simulink model "HyL"  (R2015b)
settings: Solver=ode23  StartTime=0.0  StopTime=1  FixedStep=1e-4  RelTol=1e-3  AbsTol=1e-4
undefined symbols (not defined in the file): a1, a2, Aa, Ab, b1, b2, base, beta, fv, hipassembly, In, KI, KP, Kva, Kvb, KvlkA, KvlkB, L, Lcyl, leak, lowerleg, lw_dz, pAo, pBo, ps, pt, sup1, up_dz, upperleg, V0A, V0B, wn
libraries: mblibv1 x22, simulink x6
settings Model: Creator=Toshiba  LastModifiedBy=Toshiba
settings SolverCC: ZeroCrossAlgorithm=Adaptive  SolverResetMethod=Robust
settings DataIOCC: OutputTimes=[0:1/30:100]
settings SimMechanicsCC: VisOnUpdateDiagram=on  VisDuringSimulation=on

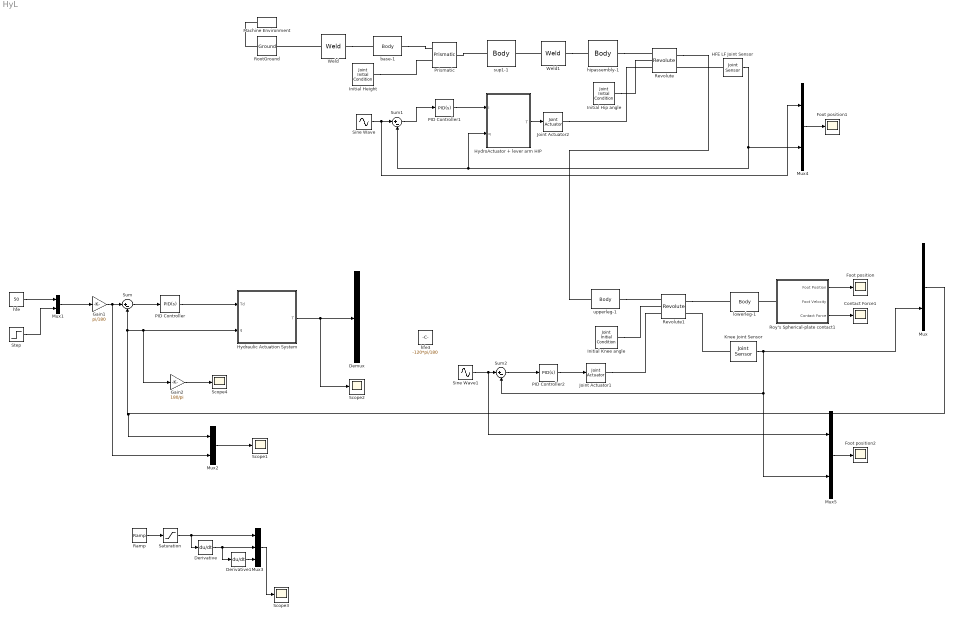
== system HyL ==
  Contact Force1 : Scope
  Demux : Demux  Outputs=2
  Derivative : Derivative
  Derivative1 : Derivative
  Foot position : Scope
  Foot position1 : Scope
  Foot position2 : Scope
  Gain1 : Gain  Gain=pi/180
  Gain2 : Gain  Gain=180/pi
  HFE LF Joint Sensor : mblibv1/Sensors &  Actuators/Joint Sensor  UpdateFromCAD=off  PhysicalDomain=Mechanical  PortType=blob  Muxed=off  Pose=off  Angle=on  AngleUnits=rad  ArcVelocity=off  ArcVelocityUnits=rad/s  ArcAcceleration=off  ArcAccelerationUnits=rad/s^2  CoordPosition=on  CoordPositionUnits=m  Velocity=off  VelocityUnits=m/s  Acceleration=off  AccelerationUnits=m/s^2  Quaternion=on  QuaternionDT=off  QuaternionDDT=off  QuaternionUnits=off  OutputVector=[ 1 ]  ActiveIO=on  Width=1  DialogClass=MechanicalSensorBlock  Primitive=R1  Force=off  ForceUnits=N  Torque=off  TorqueUnits=N*m  ReferenceFrame=Absolute (INERTIAL)  ReactionSensedSide=Base  ReactionReferenceFrame=Absolute (World)  ReactionForce=off  ReactionForceUnits=N  ReactionMoment=off  ReactionMomentUnits=N*m
  Hydraulic Actuation System : Subsystem
  HydroActuator + lever arm HIP : Subsystem
  Initial Height : mblibv1/Sensors &  Actuators/Joint Initial Condition  UpdateFromCAD=off  LeftPortType=blob  RightPortType=blob  PhysicalDomain=Mechanical  DialogClass=InitialConditionBlock  InitialConditions=P1$true$0$m$rad$0$m/s$rad/s#P2$false$0$m$rad$0$m/s$rad/s#P3$false$0$m$rad$0$m/s$rad/s#R1$false$0$m$rad$0$m/s$rad/s#R2$false$0$m$rad$0$m/s$rad/s#R3$false$0$m$rad$0$m/s$rad/s#S$false$0$m$rad$0$m/s$rad/s  P1PIC=0  P1VIC=0  P2PIC=0  P2VIC=0  P3PIC=0  P3VIC=0  R1PIC=0  R1VIC=0  R2PIC=0  R2VIC=0  R3PIC=0  R3VIC=0  SPIC=0  SVIC=0
  Initial Hip angle : mblibv1/Sensors &  Actuators/Joint Initial Condition  UpdateFromCAD=off  LeftPortType=blob  RightPortType=blob  PhysicalDomain=Mechanical  DialogClass=InitialConditionBlock  InitialConditions=P1$false$0.7$m$rad$0$m/s$rad/s#P2$false$0$m$rad$0$m/s$rad/s#P3$false$0$m$rad$0$m/s$rad/s#R1$true$45$m$deg$0$m/s$rad/s#R2$false$0$m$rad$0$m/s$rad/s#R3$false$0$m$rad$0$m/s$rad/s#S$false$0$m$rad$0$m/s$rad/s  P1PIC=0  P1VIC=0  P2PIC=0  P2VIC=0  P3PIC=0  P3VIC=0  R1PIC=45  R1VIC=0  R2PIC=0  R2VIC=0  R3PIC=0  R3VIC=0  SPIC=0  SVIC=0
  Initial Knee angle : mblibv1/Sensors &  Actuators/Joint Initial Condition  UpdateFromCAD=off  LeftPortType=blob  RightPortType=blob  PhysicalDomain=Mechanical  DialogClass=InitialConditionBlock  InitialConditions=P1$false$0.7$m$rad$0$m/s$rad/s#P2$false$0$m$rad$0$m/s$rad/s#P3$false$0$m$rad$0$m/s$rad/s#R1$true$-90$m$deg$0$m/s$rad/s#R2$false$0$m$rad$0$m/s$rad/s#R3$false$0$m$rad$0$m/s$rad/s#S$false$0$m$rad$0$m/s$rad/s  P1PIC=0  P1VIC=0  P2PIC=0  P2VIC=0  P3PIC=0  P3VIC=0  R1PIC=-90  R1VIC=0  R2PIC=0  R2VIC=0  R3PIC=0  R3VIC=0  SPIC=0  SVIC=0
  Joint Actuator1 : mblibv1/Sensors &  Actuators/Joint Actuator  UpdateFromCAD=off  PhysicalDomain=Mechanical  PortType=blob  ActuationStyle=Force  AngleUnits=deg  ArcVelocityUnits=deg/s  ArcAccelerationUnits=deg/s^2  CoordPositionUnits=m  VelocityUnits=m/s  AccelerationUnits=m/s^2  ForceUnits=N  TorqueUnits=N*m  ActiveIO=on  Width=1  DialogClass=MechanicalActuatorBlock  Primitive=R1  ReferenceFrame=Absolute (World)
  Joint Actuator2 : mblibv1/Sensors &  Actuators/Joint Actuator  UpdateFromCAD=off  PhysicalDomain=Mechanical  PortType=blob  ActuationStyle=Force  AngleUnits=deg  ArcVelocityUnits=deg/s  ArcAccelerationUnits=deg/s^2  CoordPositionUnits=m  VelocityUnits=m/s  AccelerationUnits=m/s^2  ForceUnits=N  TorqueUnits=N*m  ActiveIO=on  Width=1  DialogClass=MechanicalActuatorBlock  Primitive=R1  ReferenceFrame=Absolute (World)
  Knee Joint Sensor : mblibv1/Sensors &  Actuators/Joint Sensor  UpdateFromCAD=off  PhysicalDomain=Mechanical  PortType=blob  Muxed=off  Pose=off  Angle=on  AngleUnits=rad  ArcVelocity=off  ArcVelocityUnits=rad/s  ArcAcceleration=off  ArcAccelerationUnits=rad/s^2  CoordPosition=on  CoordPositionUnits=m  Velocity=off  VelocityUnits=m/s  Acceleration=off  AccelerationUnits=m/s^2  Quaternion=on  QuaternionDT=off  QuaternionDDT=off  QuaternionUnits=off  OutputVector=[ 1 ]  ActiveIO=on  Width=1  DialogClass=MechanicalSensorBlock  Primitive=R1  Force=off  ForceUnits=N  Torque=off  TorqueUnits=N*m  ReferenceFrame=Absolute (INERTIAL)  ReactionSensedSide=Base  ReactionReferenceFrame=Absolute (World)  ReactionForce=off  ReactionForceUnits=N  ReactionMoment=off  ReactionMomentUnits=N*m
  Machine Environment : mblibv1/Bodies/Machine Environment  PortType=env  PhysicalDomain=Mechanical  DialogTemplateClass=MECH.MachineEnvironment  SyncWhenCopied=off  Gravity=[0 -9.81 0]  GravityUnits=m/s^2  GravityAsSignal=off  Dimensionality=Auto-detect  AnalysisType=Forward dynamics  LinearAssemblyTolerance=1e-3  LinearAssemblyToleranceUnits=m  AngularAssemblyTolerance=1e-3  AngularAssemblyToleranceUnits=rad  ConstraintSolverType=Stabilizing  ConstraintRelTolerance=1e-4  ConstraintAbsTolerance=1e-4  UseRobustSingularityHandling=off  RedundancyAnalysisToleranceType=Automatically select tolerance  RedundancyAnalysisTolerance=1e-14  StatePerturbationType=Fixed  PerturbationSize=1e-5  VisualizeMachine=on  BodyVisualizationType=Use model default body geometries  BodyColorSelMode=Use model default  DefaultBodyColor=[1 0 0]
  Mux{,1..2,4..5} (5 alike) : Mux  Inputs=2
  Mux3 : Mux  Inputs=3
  PID Controller : simulink/Continuous/PID Controller  Controller=PID  TimeDomain=Continuous-time  SampleTime=-1  IntegratorMethod=Forward Euler  FilterMethod=Forward Euler  Form=Parallel  UseFilter=on  ControllerParametersSource=internal  P=200  I=0  D=6  N=100  InitialConditionSource=internal  InitialConditionForIntegrator=0  InitialConditionForFilter=0  ExternalReset=none  LimitOutput=off  UpperSaturationLimit=inf  LowerSaturationLimit=-inf  LinearizeAsGain=on  AntiWindupMode=none  Kb=1  TrackingMode=off  Kt=1  PParamMin=[]  PParamMax=[]  IParamMin=[]  IParamMax=[]  DParamMin=[]  DParamMax=[]  NParamMin=[]  NParamMax=[]  KbParamMin=[]  KbParamMax=[]  KtParamMin=[]  KtParamMax=[]  POutMin=[]  POutMax=[]  IOutMin=[]  IOutMax=[]  DOutMin=[]  DOutMax=[]  NOutMin=[]  NOutMax=[]  KbOutMin=[]  KbOutMax=[]  KtOutMin=[]  KtOutMax=[]  IntegratorOutMin=[]  IntegratorOutMax=[]  FilterOutMin=[]  FilterOutMax=[]  SumOutMin=[]  SumOutMax=[]  SumI1OutMin=[]  SumI1OutMax=[]  SumI2OutMin=[]  SumI2OutMax=[]  SumI3OutMin=[]  SumI3OutMax=[]  SumDOutMin=[]  SumDOutMax=[]  SaturationOutMin=[]  SaturationOutMax=[]  IntegratorContinuousStateAttributes=''  IntegratorStateMustResolveToSignalObject=off  IntegratorRTWStateStorageClass=Auto  FilterContinuousStateAttributes=''  FilterStateMustResolveToSignalObject=off  FilterRTWStateStorageClass=Auto  DifferentiatorICPrevScaledInput=0  DifferentiatorOutMin=[]  DifferentiatorOutMax=[]
  PID Controller1 : simulink/Continuous/PID Controller  Controller=PID  TimeDomain=Continuous-time  SampleTime=-1  IntegratorMethod=Forward Euler  FilterMethod=Forward Euler  Form=Parallel  UseFilter=on  ControllerParametersSource=internal  P=300  I=0  D=6  N=100  InitialConditionSource=internal  InitialConditionForIntegrator=0  InitialConditionForFilter=0  ExternalReset=none  LimitOutput=off  UpperSaturationLimit=inf  LowerSaturationLimit=-inf  LinearizeAsGain=on  AntiWindupMode=none  Kb=1  TrackingMode=off  Kt=1  PParamMin=[]  PParamMax=[]  IParamMin=[]  IParamMax=[]  DParamMin=[]  DParamMax=[]  NParamMin=[]  NParamMax=[]  KbParamMin=[]  KbParamMax=[]  KtParamMin=[]  KtParamMax=[]  POutMin=[]  POutMax=[]  IOutMin=[]  IOutMax=[]  DOutMin=[]  DOutMax=[]  NOutMin=[]  NOutMax=[]  KbOutMin=[]  KbOutMax=[]  KtOutMin=[]  KtOutMax=[]  IntegratorOutMin=[]  IntegratorOutMax=[]  FilterOutMin=[]  FilterOutMax=[]  SumOutMin=[]  SumOutMax=[]  SumI1OutMin=[]  SumI1OutMax=[]  SumI2OutMin=[]  SumI2OutMax=[]  SumI3OutMin=[]  SumI3OutMax=[]  SumDOutMin=[]  SumDOutMax=[]  SaturationOutMin=[]  SaturationOutMax=[]  IntegratorContinuousStateAttributes=''  IntegratorStateMustResolveToSignalObject=off  IntegratorRTWStateStorageClass=Auto  FilterContinuousStateAttributes=''  FilterStateMustResolveToSignalObject=off  FilterRTWStateStorageClass=Auto  DifferentiatorICPrevScaledInput=0  DifferentiatorOutMin=[]  DifferentiatorOutMax=[]
  PID Controller2 : simulink/Continuous/PID Controller  Controller=PID  TimeDomain=Continuous-time  SampleTime=-1  IntegratorMethod=Forward Euler  FilterMethod=Forward Euler  Form=Parallel  UseFilter=on  ControllerParametersSource=internal  P=300  I=0  D=6  N=100  InitialConditionSource=internal  InitialConditionForIntegrator=0  InitialConditionForFilter=0  ExternalReset=none  LimitOutput=off  UpperSaturationLimit=inf  LowerSaturationLimit=-inf  LinearizeAsGain=on  AntiWindupMode=none  Kb=1  TrackingMode=off  Kt=1  PParamMin=[]  PParamMax=[]  IParamMin=[]  IParamMax=[]  DParamMin=[]  DParamMax=[]  NParamMin=[]  NParamMax=[]  KbParamMin=[]  KbParamMax=[]  KtParamMin=[]  KtParamMax=[]  POutMin=[]  POutMax=[]  IOutMin=[]  IOutMax=[]  DOutMin=[]  DOutMax=[]  NOutMin=[]  NOutMax=[]  KbOutMin=[]  KbOutMax=[]  KtOutMin=[]  KtOutMax=[]  IntegratorOutMin=[]  IntegratorOutMax=[]  FilterOutMin=[]  FilterOutMax=[]  SumOutMin=[]  SumOutMax=[]  SumI1OutMin=[]  SumI1OutMax=[]  SumI2OutMin=[]  SumI2OutMax=[]  SumI3OutMin=[]  SumI3OutMax=[]  SumDOutMin=[]  SumDOutMax=[]  SaturationOutMin=[]  SaturationOutMax=[]  IntegratorContinuousStateAttributes=''  IntegratorStateMustResolveToSignalObject=off  IntegratorRTWStateStorageClass=Auto  FilterContinuousStateAttributes=''  FilterStateMustResolveToSignalObject=off  FilterRTWStateStorageClass=Auto  DifferentiatorICPrevScaledInput=0  DifferentiatorOutMin=[]  DifferentiatorOutMax=[]
  Prismatic : mblibv1/Joints/Prismatic  LConnTagsString=__newl0|SA1  RConnTagsString=__newr0  UpdateFromCAD=on  PMImportedID=base-1:-:sup1-1  NumSAPorts=1  CutJoint=off  MarkAsCut=off  Primitives=prismatic  PrimitiveProps=P1$World$[0,-1,0]$prismatic  DialogClass=JointBlock  P1Axis=[0,-1,0]
  Ramp : simulink/Sources/Ramp  slope=1  start=0.2  X0=45
  Revolute : mblibv1/Joints/Revolute  LConnTagsString=__newl0|SA1|SA2  RConnTagsString=__newr0|SA1  UpdateFromCAD=on  PMImportedID=hipassembly-1:-:upperleg-1  NumSAPorts=3  CutJoint=off  MarkAsCut=off  Primitives=prismatic  PrimitiveProps=R1$World$[0,0,1]$revolute  DialogClass=JointBlock  R1Axis=[0,0,1]
  Revolute1 : mblibv1/Joints/Revolute  LConnTagsString=__newl0|SA1|SA2  RConnTagsString=__newr0|SA1  UpdateFromCAD=on  PMImportedID=lowerleg-1:-:upperleg-1  NumSAPorts=3  CutJoint=off  MarkAsCut=off  Primitives=prismatic  PrimitiveProps=R1$World$[0,0,1]$revolute  DialogClass=JointBlock  R1Axis=[0,0,1]
  RootGround : mblibv1/Bodies/Ground  UpdateFromCAD=on  PMImportedID=RootGround  LeftPortType=env  RightPortType=workingframe  PhysicalDomain=Mechanical  DialogClass=GroundBlock  CoordPosition=[0,0,0]  CoordPositionUnits=m  StateVectorMgrId=5  MachineId=[5 0]  ShowEnvPort=on  ParameterChecksum=[385846261, 1263599045, 2134884544, 2976688461]  TopologyChecksum=[4069070087, 1221481650, 448546154, 1517678200]
  Roy's Spherical-plate contact1 : Subsystem
  Saturation : Saturate  UpperLimit=70  LowerLimit=45
  Scope{1..4} (4 alike) : Scope
  Sine Wave : Sin  Amplitude=50*pi/180  Bias=pi/18  SampleTime=0
  Sine Wave1 : Sin  Amplitude=-50*pi/180  Bias=-80*pi/180  SampleTime=0
  Step : Step  Before=-90  After=-100  SampleTime=0
  Sum : Sum  Inputs=|+-
  Sum1 : Sum  Inputs=|+-
  Sum2 : Sum  Inputs=|+-
  Weld : mblibv1/Joints/Weld  LConnTagsString=__newl0  RConnTagsString=__newr0  UpdateFromCAD=on  PMImportedID=HyL/RootPart:-:base-1  NumSAPorts=0  CutJoint=off  MarkAsCut=off  Primitives=weld  PrimitiveProps=W$WORLD$[0.57735,0.57735,0.57735]$weld  DialogClass=JointBlock  WAxis=[0.57735,0.57735,0.57735]
  Weld1 : mblibv1/Joints/Weld  LConnTagsString=__newl0  RConnTagsString=__newr0  UpdateFromCAD=on  PMImportedID=hipassembly-1:-:sup1-1  NumSAPorts=0  CutJoint=off  MarkAsCut=off  Primitives=weld  PrimitiveProps=W$WORLD$[0.57735,0.57735,0.57735]$weld  DialogClass=JointBlock  WAxis=[0.57735,0.57735,0.57735]
  base-1 : mblibv1/Bodies/Body  LConnTagsString=CS2  RConnTagsString=CS3  UpdateFromCAD=on  PMImportedID=base-1  DialogClass=MechanicalBodyBlock  Mass=3.01636  MassUnits=kg  InertiaUnits=kg*m^2  Inertia=[0.340331,0,0;0,0.0375412,0.0383358;0,0.0383358,0.34095]  Shape=Cylinder  ShapeDims=[1 1]  ShapeUnits=m  ShapeUse=false  Density=1  DensityUnits=kg/m^3  DensityUse=false  GraphicsMode=GFXFILE  GraphicsFileName=HyL - base-1.STL  BodyColorSelMode=COLORPALETTE  BodyColor=[0.392157;0.47451;0.635294]  AttachedToCS=CS1  CG=Right$CG$[0 0.398137 0.0520426]$WORLD$WORLD$m$[1 0 0;0 1 0;0 0 1]$3x3 Transform$rad$WORLD$false$base-1::CG(AUTOGEN)  WorkingFrames=Right$CS1$[0 0 0]$WORLD$WORLD$m$[1 0 0;0 1 0;0 0 1]$3x3 Transform$rad$WORLD$false$base-1::CS1(AUTOGEN)#Left$CS2$[0 0 0]$WORLD$WORLD$m$[1 0 0;0 1 0;0 0 1]$3x3 Transform$rad$WORLD$true$HyL/RootPart:-:base-1::base-1(AUTOGEN)#Right$CS3$[-0.03 1 0]$WORLD$WORLD$m$[1 0 0;0 1 0;0 0 1]$3x3 Transform$rad$WORLD$true$base-1:-:sup1-1::base-1(AUTOGEN)  CGPos=[0 0.398137 0.0520426]  CGRot=[1 0 0;0 1 0;0 0 1]  CS0Pos=[]  CS0Rot=[]  CS1Pos=[0 0 0]  CS1Rot=[1 0 0;0 1 0;0 0 1]  CS2Pos=[0 0 0]  CS2Rot=[1 0 0;0 1 0;0 0 1]  CS3Pos=[-0.03 1 0]  CS3Rot=[1 0 0;0 1 0;0 0 1]  CS4Pos=[]  CS4Rot=[]  CS5Pos=[]  CS5Rot=[]  CS6Pos=[]  CS6Rot=[]  CS7Pos=[]  CS7Rot=[]  CS8Pos=[]  CS8Rot=[]  CS9Pos=[]  CS9Rot=[]  CS10Pos=[]  CS10Rot=[]  CS11Pos=[]  CS11Rot=[]  CS12Pos=[]  CS12Rot=[]  CS13Pos=[]  CS13Rot=[]  CS14Pos=[]  CS14Rot=[]  CS15Pos=[]  CS15Rot=[]  CS16Pos=[]  CS16Rot=[]  CS17Pos=[]  CS17Rot=[]  CS18Pos=[]  CS18Rot=[]  CS19Pos=[]  CS19Rot=[]  CS20Pos=[]  CS20Rot=[]
  hfe : Constant  Value=50
  hfe3 : Constant  Value=-120*pi/180
  hipassembly-1 : mblibv1/Bodies/Body  LConnTagsString=CS2  RConnTagsString=CS3  UpdateFromCAD=on  PMImportedID=hipassembly-1  DialogClass=MechanicalBodyBlock  Mass=0.542881  MassUnits=kg  InertiaUnits=kg*m^2  Inertia=[0.00987505,1.85018e-14,0.000388351;1.85018e-14,0.0100332,8.36483e-14;0.000388351,8.36483e-14,0.000421922]  Shape=Cylinder  ShapeDims=[1 1]  ShapeUnits=m  ShapeUse=false  Density=1  DensityUnits=kg/m^3  DensityUse=false  GraphicsMode=GFXFILE  GraphicsFileName=HyL - hipassembly-1.STL  BodyColorSelMode=COLORPALETTE  BodyColor=[1 0.84314 0]  AttachedToCS=CS1  CG=Right$CG$[-0.0346571 0.786769 0.16]$WORLD$WORLD$m$[0 0 1;-1 0 0;0 -1 0]$3x3 Transform$rad$WORLD$false$hipassembly-1::CG(AUTOGEN)  WorkingFrames=Right$CS1$[-0.167 0.795 0.19]$WORLD$WORLD$m$[0 0 1;-1 0 0;0 -1 0]$3x3 Transform$rad$WORLD$false$hipassembly-1::CS1(AUTOGEN)#Left$CS2$[0.138 0.795 0.16]$WORLD$WORLD$m$[1 0 0;0 1 0;0 0 1]$3x3 Transform$rad$WORLD$true$hipassembly-1:-:sup1-1::hipassembly-1(AUTOGEN)#Right$CS3$[-0.167 0.715 0.13]$WORLD$WORLD$m$[1 0 0;0 1 0;0 0 1]$3x3 Transform$rad$WORLD$true$hipassembly-1:-:upperleg-1::hipassembly-1(AUTOGEN)  CGPos=[-0.0346571 0.786769 0.16]  CGRot=[0 0 1;-1 0 0;0 -1 0]  CS0Pos=[]  CS0Rot=[]  CS1Pos=[-0.167 0.795 0.19]  CS1Rot=[0 0 1;-1 0 0;0 -1 0]  CS2Pos=[0.138 0.795 0.16]  CS2Rot=[1 0 0;0 1 0;0 0 1]  CS3Pos=[-0.167 0.715 0.13]  CS3Rot=[1 0 0;0 1 0;0 0 1]  CS4Pos=[]  CS4Rot=[]  CS5Pos=[]  CS5Rot=[]  CS6Pos=[]  CS6Rot=[]  CS7Pos=[]  CS7Rot=[]  CS8Pos=[]  CS8Rot=[]  CS9Pos=[]  CS9Rot=[]  CS10Pos=[]  CS10Rot=[]  CS11Pos=[]  CS11Rot=[]  CS12Pos=[]  CS12Rot=[]  CS13Pos=[]  CS13Rot=[]  CS14Pos=[]  CS14Rot=[]  CS15Pos=[]  CS15Rot=[]  CS16Pos=[]  CS16Rot=[]  CS17Pos=[]  CS17Rot=[]  CS18Pos=[]  CS18Rot=[]  CS19Pos=[]  CS19Rot=[]  CS20Pos=[]  CS20Rot=[]
  lowerleg-1 : mblibv1/Bodies/Body  LConnTagsString=CS2  RConnTagsString=CS3  UpdateFromCAD=on  PMImportedID=lowerleg-1  DialogClass=MechanicalBodyBlock  Mass=0.366637  MassUnits=kg  InertiaUnits=kg*m^2  Inertia=[0.000136482,-2.4332e-06,-1.31009e-13;-2.4332e-06,0.00435174,-4.66692e-15;-1.31009e-13,-4.66692e-15,0.00430018]  Shape=Cylinder  ShapeDims=[1 1]  ShapeUnits=m  ShapeUse=false  Density=1  DensityUnits=kg/m^3  DensityUse=false  GraphicsMode=GFXFILE  GraphicsFileName=HyL - lowerleg-1.STL  BodyColorSelMode=COLORPALETTE  BodyColor=[0.79216 0.81961 0.93333]  AttachedToCS=CS1  CG=Right$CG$[-0.167053 0.194505 0.16]$WORLD$WORLD$m$[0 1 0;-1 0 0;0 0 1]$3x3 Transform$rad$WORLD$false$lowerleg-1::CG(AUTOGEN)  WorkingFrames=Right$CS1$[-0.167 0.365 0.16]$WORLD$WORLD$m$[0 1 0;-1 0 0;0 0 1]$3x3 Transform$rad$WORLD$false$lowerleg-1::CS1(AUTOGEN)#Left$CS2$[-0.167 0.365 0.19]$WORLD$WORLD$m$[1 0 0;0 1 0;0 0 1]$3x3 Transform$rad$WORLD$true$lowerleg-1:-:upperleg-1::lowerleg-1(AUTOGEN)#Right$CS3$[-0.167 0.003 0.16]$WORLD$WORLD$m$[1 0 0;0 1 0;0 0 1]$3x3 Transform$rad$WORLD$true$none  CGPos=[-0.167053 0.194505 0.16]  CGRot=[0 1 0;-1 0 0;0 0 1]  CS0Pos=[]  CS0Rot=[]  CS1Pos=[-0.167 0.365 0.16]  CS1Rot=[0 1 0;-1 0 0;0 0 1]  CS2Pos=[-0.167 0.365 0.19]  CS2Rot=[1 0 0;0 1 0;0 0 1]  CS3Pos=[-0.167 0.003 0.16]  CS3Rot=[1 0 0;0 1 0;0 0 1]  CS4Pos=[]  CS4Rot=[]  CS5Pos=[]  CS5Rot=[]  CS6Pos=[]  CS6Rot=[]  CS7Pos=[]  CS7Rot=[]  CS8Pos=[]  CS8Rot=[]  CS9Pos=[]  CS9Rot=[]  CS10Pos=[]  CS10Rot=[]  CS11Pos=[]  CS11Rot=[]  CS12Pos=[]  CS12Rot=[]  CS13Pos=[]  CS13Rot=[]  CS14Pos=[]  CS14Rot=[]  CS15Pos=[]  CS15Rot=[]  CS16Pos=[]  CS16Rot=[]  CS17Pos=[]  CS17Rot=[]  CS18Pos=[]  CS18Rot=[]  CS19Pos=[]  CS19Rot=[]  CS20Pos=[]  CS20Rot=[]
  sup1-1 : mblibv1/Bodies/Body  LConnTagsString=CS2  RConnTagsString=CS3  UpdateFromCAD=on  PMImportedID=sup1-1  DialogClass=MechanicalBodyBlock  Mass=0.390747  MassUnits=kg  InertiaUnits=kg*m^2  Inertia=[0.000989188,0,8.1711e-05;0,0.00392443,0;8.1711e-05,0,0.00310143]  Shape=Cylinder  ShapeDims=[1 1]  ShapeUnits=m  ShapeUse=false  Density=1  DensityUnits=kg/m^3  DensityUse=false  GraphicsMode=GFXFILE  GraphicsFileName=HyL - sup1-1.STL  BodyColorSelMode=COLORPALETTE  BodyColor=[1;0.843137;0]  AttachedToCS=CS1  CG=Right$CG$[-0.00480321 0.795 0.0658853]$WORLD$WORLD$m$[-1 0 0;0 1 0;0 0 -1]$3x3 Transform$rad$WORLD$false$sup1-1::CG(AUTOGEN)  WorkingFrames=Right$CS1$[-0.1275 0.77 0.04]$WORLD$WORLD$m$[-1 0 0;0 1 0;0 0 -1]$3x3 Transform$rad$WORLD$false$sup1-1::CS1(AUTOGEN)#Left$CS2$[-0.03 0.77 0]$WORLD$WORLD$m$[1 0 0;0 1 0;0 0 1]$3x3 Transform$rad$WORLD$true$hipassembly-1:-:sup1-1::sup1-1(AUTOGEN)#Right$CS3$[0.138 0.795 0.16]$WORLD$WORLD$m$[1 0 0;0 1 0;0 0 1]$3x3 Transform$rad$WORLD$true$base-1:-:sup1-1::sup1-1(AUTOGEN)  CGPos=[-0.00480321 0.795 0.0658853]  CGRot=[-1 0 0;0 1 0;0 0 -1]  CS0Pos=[]  CS0Rot=[]  CS1Pos=[-0.1275 0.77 0.04]  CS1Rot=[-1 0 0;0 1 0;0 0 -1]  CS2Pos=[-0.03 0.77 0]  CS2Rot=[1 0 0;0 1 0;0 0 1]  CS3Pos=[0.138 0.795 0.16]  CS3Rot=[1 0 0;0 1 0;0 0 1]  CS4Pos=[]  CS4Rot=[]  CS5Pos=[]  CS5Rot=[]  CS6Pos=[]  CS6Rot=[]  CS7Pos=[]  CS7Rot=[]  CS8Pos=[]  CS8Rot=[]  CS9Pos=[]  CS9Rot=[]  CS10Pos=[]  CS10Rot=[]  CS11Pos=[]  CS11Rot=[]  CS12Pos=[]  CS12Rot=[]  CS13Pos=[]  CS13Rot=[]  CS14Pos=[]  CS14Rot=[]  CS15Pos=[]  CS15Rot=[]  CS16Pos=[]  CS16Rot=[]  CS17Pos=[]  CS17Rot=[]  CS18Pos=[]  CS18Rot=[]  CS19Pos=[]  CS19Rot=[]  CS20Pos=[]  CS20Rot=[]
  upperleg-1 : mblibv1/Bodies/Body  LConnTagsString=CS2  RConnTagsString=CS3  UpdateFromCAD=on  PMImportedID=upperleg-1  DialogClass=MechanicalBodyBlock  Mass=0.355912  MassUnits=kg  InertiaUnits=kg*m^2  Inertia=[0.000491126,-0.000103005,-2.17568e-13;-0.000103005,0.00492758,1.53749e-14;-2.17568e-13,1.53749e-14,0.00462609]  Shape=Cylinder  ShapeDims=[1 1]  ShapeUnits=m  ShapeUse=false  Density=1  DensityUnits=kg/m^3  DensityUse=false  GraphicsMode=GFXFILE  GraphicsFileName=HyL - upperleg-1.STL  BodyColorSelMode=COLORPALETTE  BodyColor=[0.466667;0.67451;0.188235]  AttachedToCS=CS1  CG=Right$CG$[-0.165551 0.545266 0.16]$WORLD$WORLD$m$[0 1 0;-1 0 0;0 0 1]$3x3 Transform$rad$WORLD$false$upperleg-1::CG(AUTOGEN)  WorkingFrames=Right$CS1$[-0.167 0.715 0.16]$WORLD$WORLD$m$[0 1 0;-1 0 0;0 0 1]$3x3 Transform$rad$WORLD$false$upperleg-1::CS1(AUTOGEN)#Left$CS2$[-0.167 0.715 0.13]$WORLD$WORLD$m$[1 0 0;0 1 0;0 0 1]$3x3 Transform$rad$WORLD$true$hipassembly-1:-:upperleg-1::upperleg-1(AUTOGEN)#Right$CS3$[-0.167 0.365 0.19]$WORLD$WORLD$m$[1 0 0;0 1 0;0 0 1]$3x3 Transform$rad$WORLD$true$lowerleg-1:-:upperleg-1::upperleg-1(AUTOGEN)  CGPos=[-0.165551 0.545266 0.16]  CGRot=[0 1 0;-1 0 0;0 0 1]  CS0Pos=[]  CS0Rot=[]  CS1Pos=[-0.167 0.715 0.16]  CS1Rot=[0 1 0;-1 0 0;0 0 1]  CS2Pos=[-0.167 0.715 0.13]  CS2Rot=[1 0 0;0 1 0;0 0 1]  CS3Pos=[-0.167 0.365 0.19]  CS3Rot=[1 0 0;0 1 0;0 0 1]  CS4Pos=[]  CS4Rot=[]  CS5Pos=[]  CS5Rot=[]  CS6Pos=[]  CS6Rot=[]  CS7Pos=[]  CS7Rot=[]  CS8Pos=[]  CS8Rot=[]  CS9Pos=[]  CS9Rot=[]  CS10Pos=[]  CS10Rot=[]  CS11Pos=[]  CS11Rot=[]  CS12Pos=[]  CS12Rot=[]  CS13Pos=[]  CS13Rot=[]  CS14Pos=[]  CS14Rot=[]  CS15Pos=[]  CS15Rot=[]  CS16Pos=[]  CS16Rot=[]  CS17Pos=[]  CS17Rot=[]  CS18Pos=[]  CS18Rot=[]  CS19Pos=[]  CS19Rot=[]  CS20Pos=[]  CS20Rot=[]
  wires:
  Roy's Spherical-plate contact1/3(Contact Force) -> Contact Force1/1
  Roy's Spherical-plate contact1/1(Foot Position) -> Foot position/1
  Mux/1 -> Mux2/1, Gain2/1, Hydraulic Actuation System/2(q), Sum/2
  Mux1/1 -> Gain1/1
  Step/1 -> Mux1/2
  hfe/1 -> Mux1/1
  Sum/1 -> PID Controller/1
  Gain1/1 -> Mux2/2, Sum/1
  PID Controller/1 -> Hydraulic Actuation System/1(Td)
  Hydraulic Actuation System/1(T) -> Scope2/1, Demux/1
  Knee Joint Sensor/1 -> Mux/2, Mux5/2, Sum2/2
  Mux2/1 -> Scope1/1
  Gain2/1 -> Scope4/1
  Derivative1/1 -> Mux3/3
  Derivative/1 -> Derivative1/1, Mux3/2
  Saturation/1 -> Derivative/1, Mux3/1
  Ramp/1 -> Saturation/1
  Mux3/1 -> Scope3/1
  Sine Wave/1 -> Mux4/1, Sum1/1
  Sum1/1 -> PID Controller1/1
  HFE LF Joint Sensor/1 -> Mux4/2, HydroActuator + lever arm HIP/2(q), Sum1/2
  Mux4/1 -> Foot position1/1
  Sine Wave1/1 -> Mux5/1, Sum2/1
  Sum2/1 -> PID Controller2/1
  PID Controller2/1 -> Joint Actuator1/1
  Mux5/1 -> Foot position2/1
  HydroActuator + lever arm HIP/1(T) -> Joint Actuator2/1
  PID Controller1/1 -> HydroActuator + lever arm HIP/1(I)
  connections:
  Weld/RConn1 -- base-1/LConn1
  hipassembly-1/RConn1 -- Revolute/LConn1
  Revolute/RConn1 -- upperleg-1/LConn1
  base-1/RConn1 -- Prismatic/LConn1
  upperleg-1/RConn1 -- Revolute1/LConn1
  Revolute1/RConn1 -- lowerleg-1/LConn1
  RootGround/LConn1 -- Machine Environment/RConn1
  Weld/LConn1 -- RootGround/RConn1
  Prismatic/RConn1 -- sup1-1/LConn1
  Roy's Spherical-plate contact1/LConn1 -- lowerleg-1/RConn1
  Weld1/LConn1 -- sup1-1/RConn1
  Weld1/RConn1 -- hipassembly-1/LConn1
  HFE LF Joint Sensor/LConn1 -- Revolute/RConn2
  Initial Knee angle/RConn1 -- Revolute1/LConn2
  Knee Joint Sensor/LConn1 -- Revolute1/RConn2
  Joint Actuator1/RConn1 -- Revolute1/LConn3
  Initial Height/RConn1 -- Prismatic/LConn2
  Initial Hip angle/RConn1 -- Revolute/LConn2
  Joint Actuator2/RConn1 -- Revolute/LConn3

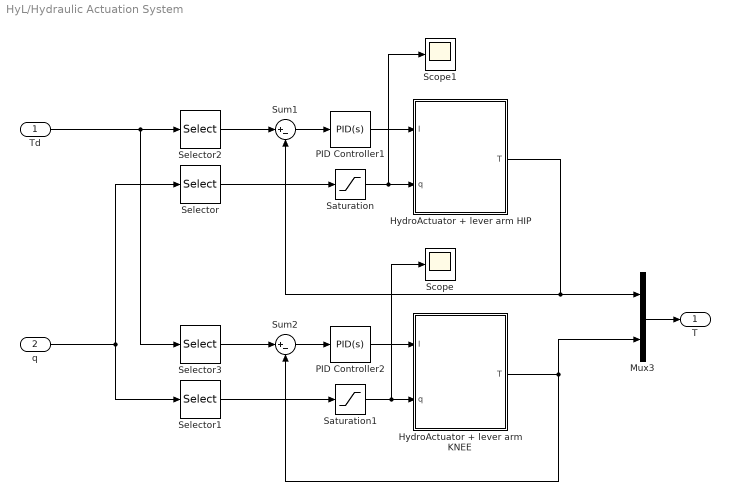
== system HyL/Hydraulic Actuation System ==
  Td : Inport
  q : Inport  Port=2
  HydroActuator + lever arm HIP : Subsystem
  HydroActuator + lever arm KNEE : Subsystem
  Mux3 : Mux  Inputs=2
  PID Controller1 : simulink/Continuous/PID Controller  Controller=PID  TimeDomain=Continuous-time  SampleTime=-1  IntegratorMethod=Forward Euler  FilterMethod=Forward Euler  Form=Parallel  UseFilter=on  ControllerParametersSource=internal  P=KP  I=KI  D=0  N=0  InitialConditionSource=internal  InitialConditionForIntegrator=0  InitialConditionForFilter=0  ExternalReset=none  LimitOutput=off  UpperSaturationLimit=inf  LowerSaturationLimit=-inf  LinearizeAsGain=on  AntiWindupMode=none  Kb=1  TrackingMode=off  Kt=1  PParamMin=[]  PParamMax=[]  IParamMin=[]  IParamMax=[]  DParamMin=[]  DParamMax=[]  NParamMin=[]  NParamMax=[]  KbParamMin=[]  KbParamMax=[]  KtParamMin=[]  KtParamMax=[]  POutMin=[]  POutMax=[]  IOutMin=[]  IOutMax=[]  DOutMin=[]  DOutMax=[]  NOutMin=[]  NOutMax=[]  KbOutMin=[]  KbOutMax=[]  KtOutMin=[]  KtOutMax=[]  IntegratorOutMin=[]  IntegratorOutMax=[]  FilterOutMin=[]  FilterOutMax=[]  SumOutMin=[]  SumOutMax=[]  SumI1OutMin=[]  SumI1OutMax=[]  SumI2OutMin=[]  SumI2OutMax=[]  SumI3OutMin=[]  SumI3OutMax=[]  SumDOutMin=[]  SumDOutMax=[]  SaturationOutMin=[]  SaturationOutMax=[]  IntegratorContinuousStateAttributes=''  IntegratorStateMustResolveToSignalObject=off  IntegratorRTWStateStorageClass=Auto  FilterContinuousStateAttributes=''  FilterStateMustResolveToSignalObject=off  FilterRTWStateStorageClass=Auto  DifferentiatorICPrevScaledInput=0  DifferentiatorOutMin=[]  DifferentiatorOutMax=[]
  PID Controller2 : simulink/Continuous/PID Controller  Controller=PID  TimeDomain=Continuous-time  SampleTime=-1  IntegratorMethod=Forward Euler  FilterMethod=Forward Euler  Form=Parallel  UseFilter=on  ControllerParametersSource=internal  P=KP  I=KI  D=0  N=0  InitialConditionSource=internal  InitialConditionForIntegrator=0  InitialConditionForFilter=0  ExternalReset=none  LimitOutput=off  UpperSaturationLimit=inf  LowerSaturationLimit=-inf  LinearizeAsGain=on  AntiWindupMode=none  Kb=1  TrackingMode=off  Kt=1  PParamMin=[]  PParamMax=[]  IParamMin=[]  IParamMax=[]  DParamMin=[]  DParamMax=[]  NParamMin=[]  NParamMax=[]  KbParamMin=[]  KbParamMax=[]  KtParamMin=[]  KtParamMax=[]  POutMin=[]  POutMax=[]  IOutMin=[]  IOutMax=[]  DOutMin=[]  DOutMax=[]  NOutMin=[]  NOutMax=[]  KbOutMin=[]  KbOutMax=[]  KtOutMin=[]  KtOutMax=[]  IntegratorOutMin=[]  IntegratorOutMax=[]  FilterOutMin=[]  FilterOutMax=[]  SumOutMin=[]  SumOutMax=[]  SumI1OutMin=[]  SumI1OutMax=[]  SumI2OutMin=[]  SumI2OutMax=[]  SumI3OutMin=[]  SumI3OutMax=[]  SumDOutMin=[]  SumDOutMax=[]  SaturationOutMin=[]  SaturationOutMax=[]  IntegratorContinuousStateAttributes=''  IntegratorStateMustResolveToSignalObject=off  IntegratorRTWStateStorageClass=Auto  FilterContinuousStateAttributes=''  FilterStateMustResolveToSignalObject=off  FilterRTWStateStorageClass=Auto  DifferentiatorICPrevScaledInput=0  DifferentiatorOutMin=[]  DifferentiatorOutMax=[]
  Saturation : Saturate  UpperLimit=70*pi/180  LowerLimit=-50*pi/180
  Saturation1 : Saturate  UpperLimit=-20*pi/180  LowerLimit=-140*pi/180
  Scope : Scope
  Scope1 : Scope
  Selector : Selector  InputPortWidth=2  IndexOptions=Index vector (dialog)  Indices=1  OutputSizes=1
  Selector1 : Selector  InputPortWidth=2  IndexOptions=Index vector (dialog)  Indices=2  OutputSizes=1
  Selector2 : Selector  InputPortWidth=2  IndexOptions=Index vector (dialog)  Indices=1  OutputSizes=1
  Selector3 : Selector  InputPortWidth=2  IndexOptions=Index vector (dialog)  Indices=2  OutputSizes=1
  Sum1 : Sum  Inputs=|+-
  Sum2 : Sum  Inputs=|+-
  T : Outport
  wires:
  PID Controller1/1 -> HydroActuator + lever arm HIP/1(I)
  Sum1/1 -> PID Controller1/1
  HydroActuator + lever arm HIP/1(T) -> Sum1/2, Mux3/1
  Selector/1 -> Saturation/1
  Selector2/1 -> Sum1/1
  Sum2/1 -> PID Controller2/1
  Selector1/1 -> Saturation1/1
  Selector3/1 -> Sum2/1
  PID Controller2/1 -> HydroActuator + lever arm KNEE/1(I)
  HydroActuator + lever arm KNEE/1(T) -> Sum2/2, Mux3/2
  Mux3/1 -> T/1
  q/1 -> Selector1/1, Selector/1
  Td/1 -> Selector2/1, Selector3/1
  Saturation/1 -> Scope1/1, HydroActuator + lever arm HIP/2(q)
  Saturation1/1 -> Scope/1, HydroActuator + lever arm KNEE/2(q)

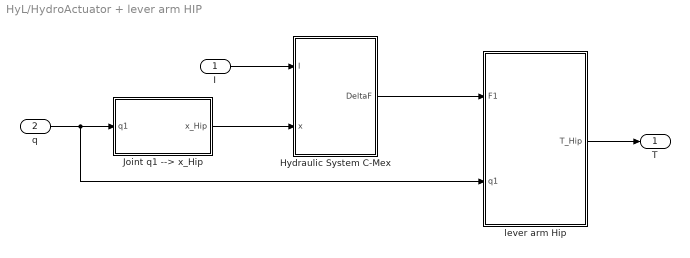
== system HyL/HydroActuator + lever arm HIP ==
  I : Inport
  q : Inport  Port=2
  Hydraulic System C-Mex : Subsystem
  "Joint q1 --> x_Hip  " : MATLAB Function  TreatAsAtomicUnit=on
  lever arm Hip : MATLAB Function  TreatAsAtomicUnit=on
  T : Outport
  wires:
  q/1 -> "Joint q1 --> x_Hip  "/1(q1), lever arm Hip/2(q1)
  lever arm Hip/1(T_Hip) -> T/1
  Hydraulic System C-Mex/1(DeltaF) -> lever arm Hip/1(F1)
  "Joint q1 --> x_Hip  "/1(x_Hip) -> Hydraulic System C-Mex/2(x)
  I/1 -> Hydraulic System C-Mex/1(I)

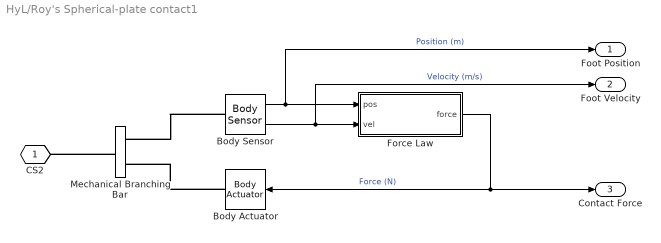
== system HyL/Roy's Spherical-plate contact1 ==
  Body Actuator : mblibv1/Sensors &  Actuators/Body Actuator  UpdateFromCAD=off  PhysicalDomain=Mechanical  PortType=blob  ActuationStyle=Force  AngleUnits=deg  ArcVelocityUnits=deg/s  ArcAccelerationUnits=deg/s^2  CoordPositionUnits=m  VelocityUnits=m/s  AccelerationUnits=m/s^2  ForceUnits=N  TorqueUnits=N*m  ActiveIO=on  Width=3  DialogClass=MechanicalActuatorBlock  ReferenceFrame=Absolute (World)  Angle=off  CoordPosition=on  Force=on  Torque=off
  Body Sensor : mblibv1/Sensors &  Actuators/Body Sensor  UpdateFromCAD=off  PhysicalDomain=Mechanical  PortType=blob  Muxed=off  Pose=off  Angle=on  AngleUnits=deg  ArcVelocity=off  ArcVelocityUnits=deg/s  ArcAcceleration=off  ArcAccelerationUnits=deg/s^2  CoordPosition=on  CoordPositionUnits=m  Velocity=on  VelocityUnits=m/s  Acceleration=off  AccelerationUnits=m/s^2  Quaternion=on  QuaternionDT=off  QuaternionDDT=off  QuaternionUnits=off  OutputVector=[ 3 3 ]  ActiveIO=on  Width=6  DialogClass=MechanicalSensorBlock  ReferenceFrame=Absolute (World)
  Force Law : Subsystem
  Mechanical Branching Bar : mblibv1/Utilities/Mechanical Branching Bar  LConnTagsString=_newl0  RConnTagsString=SA0|SA1  UpdateFromCAD=off  DialogClass=MechanicalBranchingBarBlock  NumSAPorts=2
  CS2 : PMIOPort  Tag=PMCPort  Port=1  Side=Left
  Foot Position : Outport
  Foot Velocity : Outport  Port=2
  Contact Force : Outport  Port=3
  wires:
  Body Sensor/1 -> Force Law/1(pos), Foot Position/1  "Position (m)"
  Body Sensor/2 -> Force Law/2(vel), Foot Velocity/1  "Velocity (m/s)"
  Force Law/1(force) -> Body Actuator/1, Contact Force/1  "Force (N)"
  connections:
  Mechanical Branching Bar/LConn1 -- CS2/RConn1
  Body Actuator/RConn1 -- Mechanical Branching Bar/RConn2
  Body Sensor/LConn1 -- Mechanical Branching Bar/RConn1

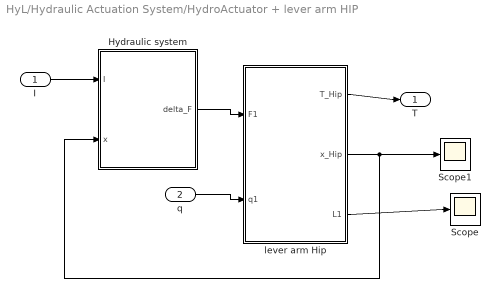
== system HyL/Hydraulic Actuation System/HydroActuator + lever arm HIP ==
  I : Inport
  q : Inport  Port=2
  Hydraulic system : Subsystem
  Scope : Scope
  Scope1 : Scope
  lever arm Hip : MATLAB Function  TreatAsAtomicUnit=on
  T : Outport
  wires:
  Hydraulic system/1(delta_F) -> lever arm Hip/1(F1)
  lever arm Hip/1(T_Hip) -> T/1
  I/1 -> Hydraulic system/1(I)
  q/1 -> lever arm Hip/2(q1)
  lever arm Hip/2(x_Hip) -> Scope1/1, Hydraulic system/2(x)
  lever arm Hip/3(L1) -> Scope/1

== system HyL/Hydraulic Actuation System/HydroActuator + lever arm KNEE ==
  I : Inport
  q : Inport  Port=2
  Hydraulic system : Subsystem
  lever arm Knee : MATLAB Function  TreatAsAtomicUnit=on
  T : Outport
  wires:
  q/1 -> lever arm Knee/2(q2)
  lever arm Knee/2(x_Knee) -> Hydraulic system/2(x)
  Hydraulic system/1(delta_F) -> lever arm Knee/1(F2)
  I/1 -> Hydraulic system/1(I)
  lever arm Knee/1(T_Knee) -> T/1

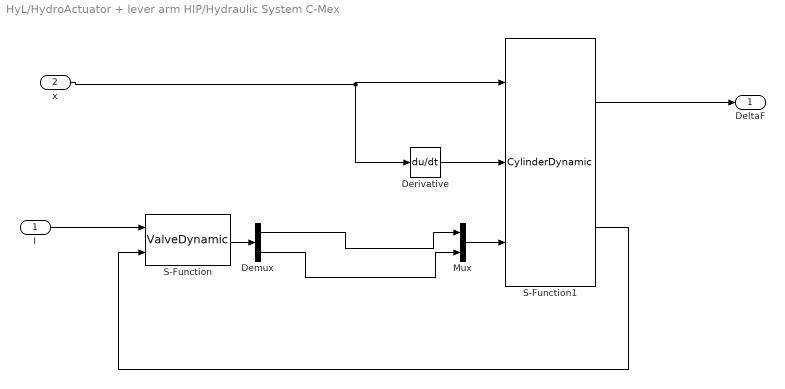
== system HyL/HydroActuator + lever arm HIP/Hydraulic System C-Mex ==
  I : Inport
  x : Inport  Port=2
  Demux : Demux  Outputs=2
  Derivative : Derivative
  Mux : Mux  Inputs=2
  S-Function : S-Function  FunctionName=ValveDynamic  Parameters=wn, E, In, Kva, Kvb, KvlkA, KvlkB, ps, pt,up_dz,lw_dz  SFunctionDeploymentMode=off  EnableBusSupport=off
  S-Function1 : S-Function  FunctionName=CylinderDynamic  Parameters=beta, V0A, V0B, Aa, Ab, L, fv, leak  SFunctionDeploymentMode=off  EnableBusSupport=off
  DeltaF : Outport
  wires:
  I/1 -> S-Function/1
  Derivative/1 -> S-Function1/2
  x/1 -> S-Function1/1, Derivative/1
  S-Function1/1 -> DeltaF/1
  S-Function1/2 -> S-Function/2
  S-Function/1 -> Demux/1
  Mux/1 -> S-Function1/3
  Demux/2 -> Mux/2
  Demux/1 -> Mux/1

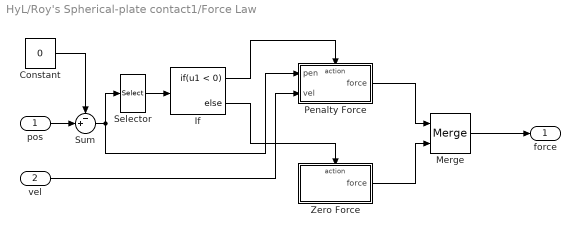
== system HyL/Roy's Spherical-plate contact1/Force Law ==
  pos : Inport
  vel : Inport  Port=2
  Constant : Constant  Value=0
  If : If  IfExpression=u1 < 0
  Merge : Merge  InitialOutput=0  InputPortOffsets=0
  Penalty Force : Subsystem  TreatAsAtomicUnit=on
  Selector : Selector  InputPortWidth=3  IndexOptions=Index vector (dialog)  Indices=[2]  OutputSizes=1
  Sum : Sum  Inputs=-+|  SaturateOnIntegerOverflow=on
  Zero Force : Subsystem  TreatAsAtomicUnit=on
  force : Outport
  wires:
  pos/1 -> Sum/2
  Sum/1 -> Penalty Force/1(pen), Selector/1
  Constant/1 -> Sum/1
  vel/1 -> Penalty Force/2(vel)
  If/2 -> Zero Force/Action
  Penalty Force/1(force) -> Merge/1
  Zero Force/1(force) -> Merge/2
  Merge/1 -> force/1
  If/1 -> Penalty Force/Action
  Selector/1 -> If/1

== system HyL/Hydraulic Actuation System/HydroActuator + lever arm HIP/Hydraulic system ==
  I : Inport
  x : Inport  Port=2
  Cylinder HOERBIGER LB6 1610 0080 4M : Subsystem
  Servovalve MOOG E024-177LA : Subsystem
  delta_F : Outport
  wires:
  Servovalve MOOG E024-177LA/2(qB) -> Cylinder HOERBIGER LB6 1610 0080 4M/2(qB)
  Servovalve MOOG E024-177LA/1(qA) -> Cylinder HOERBIGER LB6 1610 0080 4M/1(qA)
  Cylinder HOERBIGER LB6 1610 0080 4M/2(pA1) -> Servovalve MOOG E024-177LA/2(pA)
  Cylinder HOERBIGER LB6 1610 0080 4M/3(pB1) -> Servovalve MOOG E024-177LA/3(pB)
  I/1 -> Servovalve MOOG E024-177LA/1(I)
  Cylinder HOERBIGER LB6 1610 0080 4M/1(delta_F) -> delta_F/1
  x/1 -> Cylinder HOERBIGER LB6 1610 0080 4M/3(x)

== system HyL/Hydraulic Actuation System/HydroActuator + lever arm KNEE/Hydraulic system ==
  I : Inport
  x : Inport  Port=2
  Cylinder HOERBIGER LB6 1610 0080 4M : Subsystem
  Servovalve MOOG E024-177LA : Subsystem
  delta_F : Outport
  wires:
  Servovalve MOOG E024-177LA/2(qB) -> Cylinder HOERBIGER LB6 1610 0080 4M/2(qB)
  Servovalve MOOG E024-177LA/1(qA) -> Cylinder HOERBIGER LB6 1610 0080 4M/1(qA)
  Cylinder HOERBIGER LB6 1610 0080 4M/2(pA1) -> Servovalve MOOG E024-177LA/2(pA)
  Cylinder HOERBIGER LB6 1610 0080 4M/3(pB1) -> Servovalve MOOG E024-177LA/3(pB)
  I/1 -> Servovalve MOOG E024-177LA/1(I)
  Cylinder HOERBIGER LB6 1610 0080 4M/1(delta_F) -> delta_F/1
  x/1 -> Cylinder HOERBIGER LB6 1610 0080 4M/3(x)

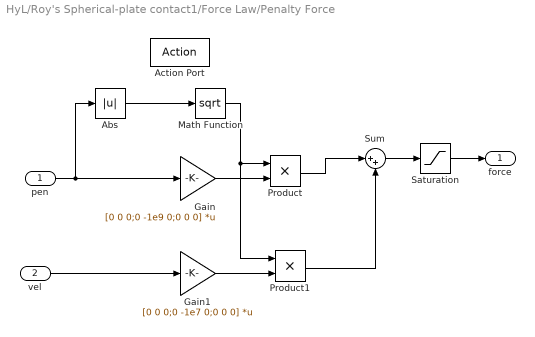
== system HyL/Roy's Spherical-plate contact1/Force Law/Penalty Force ==
  pen : Inport
  vel : Inport  Port=2
  Action Port : ActionPort  ActionType=then
  Abs : Abs  ZeroCross=off
  Gain : Gain  Gain=[0 0 0;0 -1e9 0;0 0 0]  Multiplication=Matrix(K*u)  SaturateOnIntegerOverflow=on  OutDataTypeStr=Inherit: Same as input  ParamDataTypeStr=Inherit: Same as input
  Gain1 : Gain  Gain=[0 0 0;0 -1e7 0;0 0 0]  Multiplication=Matrix(K*u)  SaturateOnIntegerOverflow=on  OutDataTypeStr=Inherit: Same as input  ParamDataTypeStr=Inherit: Same as input
  Math Function : Math  Operator=sqrt  SaturateOnIntegerOverflow=on
  Product : Product  RndMeth=Zero
  Product1 : Product  RndMeth=Zero
  Saturation : Saturate  UpperLimit=inf  LowerLimit=0
  Sum : Sum  Inputs=|++  SaturateOnIntegerOverflow=on
  force : Outport  InitialOutput=0
  wires:
  pen/1 -> Gain/1, Abs/1
  Sum/1 -> Saturation/1
  vel/1 -> Gain1/1
  Saturation/1 -> force/1
  Abs/1 -> Math Function/1
  Math Function/1 -> Product/1, Product1/1
  Gain/1 -> Product/2
  Product/1 -> Sum/1
  Product1/1 -> Sum/2
  Gain1/1 -> Product1/2

== system HyL/Roy's Spherical-plate contact1/Force Law/Zero Force ==
  Action Port : ActionPort  ActionType=else
  Zero Force : Constant  Value=[0;0;0]
  force : Outport  InitialOutput=0
  wires:
  Zero Force/1 -> force/1

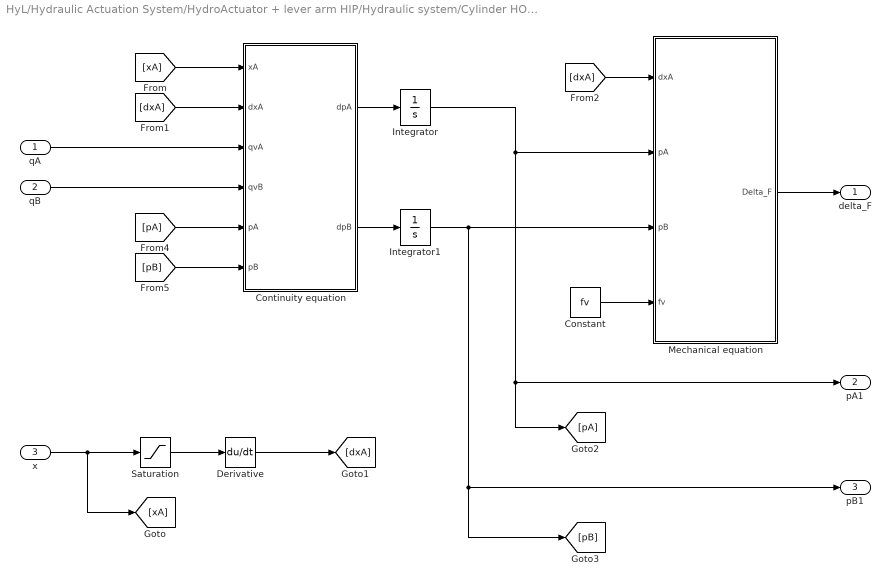
== system HyL/Hydraulic Actuation System/HydroActuator + lever arm HIP/Hydraulic system/Cylinder HOERBIGER LB6 1610 0080 4M ==
  qA : Inport
  qB : Inport  Port=2
  x : Inport  Port=3
  Constant : Constant  Value=fv
  Continuity equation : MATLAB Function  TreatAsAtomicUnit=on
  Derivative : Derivative
  Integrator : Integrator  InitialCondition=pAo
  Integrator1 : Integrator  InitialCondition=pBo
  Mechanical equation : MATLAB Function  TreatAsAtomicUnit=on
  Saturation : Saturate  UpperLimit=L  LowerLimit=0
  delta_F : Outport
  pA1 : Outport  Port=2
  pB1 : Outport  Port=3
  wires:
  Continuity equation/1(dpA) -> Integrator/1
  Continuity equation/2(dpB) -> Integrator1/1
  qA/1 -> Continuity equation/3(qvA)
  qB/1 -> Continuity equation/4(qvB)
  [dxA] -> Continuity equation/2(dxA)
  [xA] -> Continuity equation/1(xA)
  Constant/1 -> Mechanical equation/4(fv)
  Derivative/1 -> [dxA]
  Mechanical equation/1(Delta_F) -> delta_F/1
  x/1 -> [xA], Saturation/1
  Saturation/1 -> Derivative/1
  [dxA] -> Mechanical equation/1(dxA)
  Integrator/1 -> [pA], pA1/1, Mechanical equation/2(pA)
  Integrator1/1 -> [pB], pB1/1, Mechanical equation/3(pB)
  [pA] -> Continuity equation/5(pA)
  [pB] -> Continuity equation/6(pB)

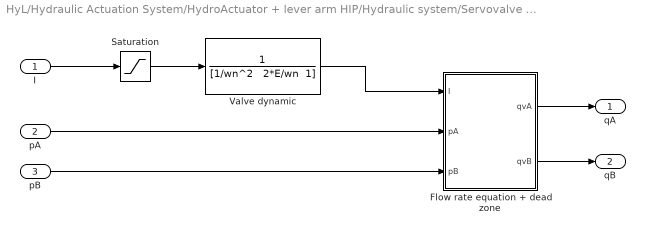
== system HyL/Hydraulic Actuation System/HydroActuator + lever arm HIP/Hydraulic system/Servovalve MOOG E024-177LA ==
  I : Inport
  pA : Inport  Port=2
  pB : Inport  Port=3
  Flow rate equation + dead zone : MATLAB Function  TreatAsAtomicUnit=on
  Saturation : Saturate  UpperLimit=In  LowerLimit=-In  LinearizeAsGain=off
  Valve dynamic : TransferFcn  Numerator=1  Denominator="[1/wn^2   2*E/wn  1]"
  qA : Outport
  qB : Outport  Port=2
  wires:
  Saturation/1 -> Valve dynamic/1
  I/1 -> Saturation/1
  Valve dynamic/1 -> Flow rate equation + dead zone/1(I)
  pA/1 -> Flow rate equation + dead zone/2(pA)
  pB/1 -> Flow rate equation + dead zone/3(pB)
  Flow rate equation + dead zone/2(qvB) -> qB/1
  Flow rate equation + dead zone/1(qvA) -> qA/1

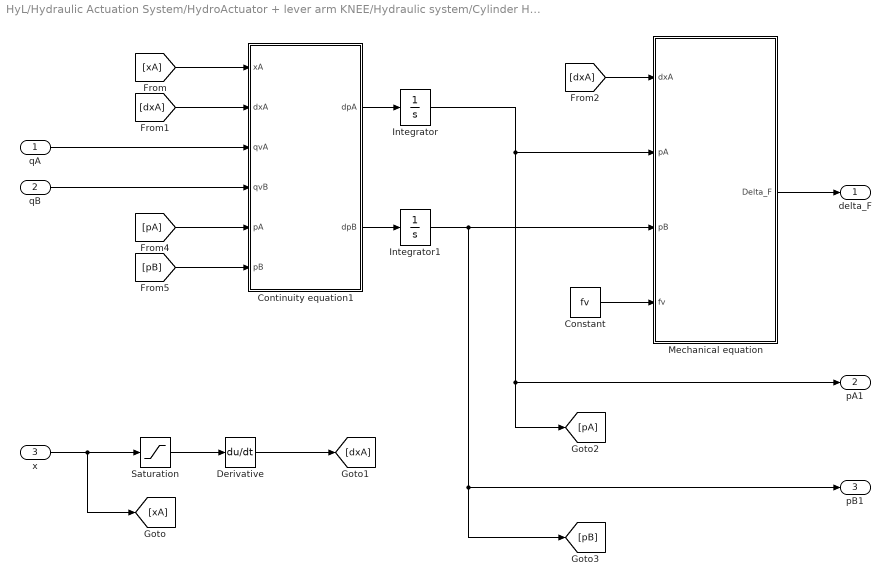
== system HyL/Hydraulic Actuation System/HydroActuator + lever arm KNEE/Hydraulic system/Cylinder HOERBIGER LB6 1610 0080 4M ==
  qA : Inport
  qB : Inport  Port=2
  x : Inport  Port=3
  Constant : Constant  Value=fv
  Continuity equation1 : MATLAB Function  TreatAsAtomicUnit=on
  Derivative : Derivative
  Integrator : Integrator  InitialCondition=pAo
  Integrator1 : Integrator  InitialCondition=pBo
  Mechanical equation : MATLAB Function  TreatAsAtomicUnit=on
  Saturation : Saturate  UpperLimit=L  LowerLimit=0
  delta_F : Outport
  pA1 : Outport  Port=2
  pB1 : Outport  Port=3
  wires:
  Continuity equation1/1(dpA) -> Integrator/1
  Continuity equation1/2(dpB) -> Integrator1/1
  qA/1 -> Continuity equation1/3(qvA)
  qB/1 -> Continuity equation1/4(qvB)
  [dxA] -> Continuity equation1/2(dxA)
  [xA] -> Continuity equation1/1(xA)
  Constant/1 -> Mechanical equation/4(fv)
  Derivative/1 -> [dxA]
  Mechanical equation/1(Delta_F) -> delta_F/1
  x/1 -> [xA], Saturation/1
  Saturation/1 -> Derivative/1
  [dxA] -> Mechanical equation/1(dxA)
  Integrator/1 -> [pA], pA1/1, Mechanical equation/2(pA)
  Integrator1/1 -> [pB], pB1/1, Mechanical equation/3(pB)
  [pA] -> Continuity equation1/5(pA)
  [pB] -> Continuity equation1/6(pB)

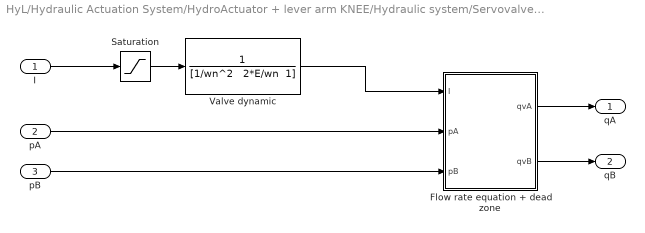
== system HyL/Hydraulic Actuation System/HydroActuator + lever arm KNEE/Hydraulic system/Servovalve MOOG E024-177LA ==
  I : Inport
  pA : Inport  Port=2
  pB : Inport  Port=3
  Flow rate equation + dead zone : MATLAB Function  TreatAsAtomicUnit=on
  Saturation : Saturate  UpperLimit=In  LowerLimit=-In  LinearizeAsGain=off
  Valve dynamic : TransferFcn  Numerator=1  Denominator="[1/wn^2   2*E/wn  1]"
  qA : Outport
  qB : Outport  Port=2
  wires:
  Saturation/1 -> Valve dynamic/1
  I/1 -> Saturation/1
  Valve dynamic/1 -> Flow rate equation + dead zone/1(I)
  pA/1 -> Flow rate equation + dead zone/2(pA)
  pB/1 -> Flow rate equation + dead zone/3(pB)
  Flow rate equation + dead zone/2(qvB) -> qB/1
  Flow rate equation + dead zone/1(qvA) -> qA/1

== matlab function HyL/Hydraulic Actuation System/HydroActuator + lever arm KNEE/Hydraulic system/Cylinder HOERBIGER LB6 1610 0080 4M/Continuity equation1 ==
  data: xA input; dpA output; dpB output; dxA input; qvA input; qvB input; pA input; pB input; leak parameter; V0A parameter; V0B parameter; Aa parameter; Ab parameter; L parameter; beta parameter
function [dpA,dpB] = fcn(xA, dxA, qvA, qvB, pA, pB, leak, V0A, V0B, Aa, Ab, L, beta)

pC = pA - pB;   % Pressao de carga [Pa]
qvlk = leak * pC;
dpA = (beta/(V0A + Aa*xA)) * (qvA - Aa*dxA - qvlk);
dpB = (beta/(V0B + Ab*(L-xA))) * (Ab*dxA + qvlk - qvB);

== matlab function HyL/Hydraulic Actuation System/HydroActuator + lever arm HIP/Hydraulic system/Cylinder HOERBIGER LB6 1610 0080 4M/Continuity equation ==
  data: xA input; dpA output; dpB output; dxA input; qvA input; qvB input; pA input; pB input; leak parameter; V0A parameter; V0B parameter; Aa parameter; Ab parameter; L parameter; beta parameter
function [dpA,dpB] = fcn(xA, dxA, qvA, qvB, pA, pB, leak, V0A, V0B, Aa, Ab, L, beta)

pC = pA - pB;   % Pressao de carga [Pa]
qvlk = leak * pC;
dpA = (beta/(V0A + Aa*xA)) * (qvA - Aa*dxA - qvlk);
dpB = (beta/(V0B + Ab*(L-xA))) * (Ab*dxA + qvlk - qvB);

== matlab function HyL/Hydraulic Actuation System/HydroActuator + lever arm HIP/Hydraulic system/Cylinder HOERBIGER LB6 1610 0080 4M/Mechanical equation ==
  data: Delta_F output; dxA input; pA input; pB input; fv input; Aa parameter; Ab parameter
function Delta_F = fcn(dxA, pA, pB, fv, Aa, Ab)
%#codegen

FH  = pA*Aa - pB*Ab;     % N - Hydraulic force
Ffr = fv*dxA;            % N - Friction force (Viscous)
Delta_F  = FH - Ffr;     % m/s2 - Acceleration

== matlab function HyL/Hydraulic Actuation System/HydroActuator + lever arm HIP/Hydraulic system/Servovalve MOOG E024-177LA/Flow rate equation + dead zone ==
  data I settings: updateMethod=SF_CONTINUOUS_TIME_DATA
  data qvA settings: updateMethod=SF_CONTINUOUS_TIME_DATA
  data qvB settings: updateMethod=SF_CONTINUOUS_TIME_DATA
  data: I input; qvA output; qvB output; In parameter; Kva parameter; Kvb parameter; KvlkA parameter; KvlkB parameter; up_dz parameter; lw_dz parameter; ps parameter; pt parameter; pA input; pB input
function [qvA , qvB] = fcn(I, In, Kva, Kvb, KvlkA, KvlkB,up_dz, lw_dz, ps, pt, pA, pB)

if (I>=up_dz) && (I<=In),
    qvA = (Kva*(I/In) + KvlkA) * sign(ps-pA)*sqrt(abs(ps-pA)) - KvlkA*sign(pA-pt)*sqrt(abs(pA-pt)) ;
    qvB = (Kvb*(I/In) + KvlkB) * sign(pB-pt)*sqrt(abs(pB-pt)) - KvlkB*sign(ps-pB)*sqrt(abs(ps-pB)) ;
elseif (I>=-In) && (I<=lw_dz), 
    qvA = KvlkA*sign(ps-pA)*sqrt(abs(ps-pA)) - (Kva*(abs(I)/In) + KvlkA) * sign(pA-pt)*sqrt(abs(pA-pt));
     qvB = KvlkB*sign(pB-pt)*sqrt(abs(pB-pt)) - (Kvb*(abs(I)/In) + KvlkB) * sign(ps-pB)*sqrt(abs(ps-pB));
else
    qvA = 0;
    qvB = 0;
end
end

== matlab function HyL/Hydraulic Actuation System/HydroActuator + lever arm KNEE/Hydraulic system/Cylinder HOERBIGER LB6 1610 0080 4M/Mechanical equation ==
  data: Delta_F output; dxA input; pA input; pB input; fv input; Aa parameter; Ab parameter
function Delta_F = fcn(dxA, pA, pB, fv, Aa, Ab)
%#codegen

FH  = pA*Aa - pB*Ab;     % N - Hydraulic force
Ffr = fv*dxA;            % N - Friction force (Viscous)
Delta_F  = FH - Ffr;     % m/s2 - Acceleration

== matlab function HyL/Hydraulic Actuation System/HydroActuator + lever arm KNEE/Hydraulic system/Servovalve MOOG E024-177LA/Flow rate equation + dead zone ==
  data I settings: updateMethod=SF_CONTINUOUS_TIME_DATA
  data qvA settings: updateMethod=SF_CONTINUOUS_TIME_DATA
  data qvB settings: updateMethod=SF_CONTINUOUS_TIME_DATA
  data: I input; qvA output; qvB output; In parameter; Kva parameter; Kvb parameter; KvlkA parameter; KvlkB parameter; up_dz parameter; lw_dz parameter; ps parameter; pt parameter; pA input; pB input
function [qvA , qvB] = fcn(I, In, Kva, Kvb, KvlkA, KvlkB,up_dz, lw_dz, ps, pt, pA, pB)

if (I>=up_dz) && (I<=In),
    qvA = (Kva*(I/In) + KvlkA) * sign(ps-pA)*sqrt(abs(ps-pA)) - KvlkA*sign(pA-pt)*sqrt(abs(pA-pt)) ;
    qvB = (Kvb*(I/In) + KvlkB) * sign(pB-pt)*sqrt(abs(pB-pt)) - KvlkB*sign(ps-pB)*sqrt(abs(ps-pB)) ;
elseif (I>=-In) && (I<=lw_dz), 
    qvA = KvlkA*sign(ps-pA)*sqrt(abs(ps-pA)) - (Kva*(abs(I)/In) + KvlkA) * sign(pA-pt)*sqrt(abs(pA-pt));
     qvB = KvlkB*sign(pB-pt)*sqrt(abs(pB-pt)) - (Kvb*(abs(I)/In) + KvlkB) * sign(ps-pB)*sqrt(abs(ps-pB));
else
    qvA = 0;
    qvB = 0;
end
end

== matlab function HyL/Hydraulic Actuation System/HydroActuator + lever arm HIP/lever arm Hip ==
  data: a1 parameter; T_Hip output; b1 parameter; e11 parameter; e12 parameter; F1 input; Lcyl parameter; q1 input; x_Hip output; L1 output
function [T_Hip, x_Hip,L1] = fcn(a1,b1,e11,e12,F1,Lcyl,q1)
%#codegen

%Hip
ang1 = pi/2 - q1 + e11 - e12; 
c1 = sqrt(a1^2 + b1^2 - 2*a1*b1*cos(ang1));
L1 = a1*sin(acos((a1^2+c1^2-b1^2)/(2*a1*c1)));

% Outputs
T_Hip = F1*L1;
x_Hip = c1-Lcyl;

== matlab function HyL/Hydraulic Actuation System/HydroActuator + lever arm KNEE/lever arm Knee ==
  data: a2 parameter; T_Knee output; b2 parameter; e21 parameter; e22 parameter; F2 input; Lcyl parameter; q2 input; x_Knee output
function [T_Knee, x_Knee] = fcn(a2,b2,e21,e22,F2,Lcyl,q2)
%#codegen

%Knee
ang2 = pi + q2 - e21 - e22;
c2 = sqrt(a2^2 + b2^2 - 2*a2*b2*cos(ang2));
L2 = a2*sin(acos((a2^2+c2^2-b2^2)/(2*a2*c2)));

% Outputs
T_Knee = F2*L2;
x_Knee = c2-Lcyl;

== matlab function HyL/HydroActuator + lever arm HIP/Joint q1 --> x_Hip   ==
  data: a1 parameter; x_Hip output; b1 parameter; e11 parameter; e12 parameter; Lcyl parameter; q1 input
function x_Hip = fcn(a1,b1,e11,e12,Lcyl,q1)
%#codegen

%Hip
ang1 = pi/2 - q1 + e11 - e12; 
c1 = sqrt(a1^2 + b1^2 - 2*a1*b1*cos(ang1));

x_Hip = c1-Lcyl;

== matlab function HyL/HydroActuator + lever arm HIP/lever arm Hip ==
  data: a1 parameter; T_Hip output; b1 parameter; e11 parameter; e12 parameter; F1 input; q1 input
function T_Hip = fcn(a1,b1,e11,e12,F1,q1)
%#codegen

%Hip
ang1 = pi/2 - q1 + e11 - e12; 
c1 = sqrt(a1^2 + b1^2 - 2*a1*b1*cos(ang1));
L1 = a1*sin(acos((a1^2+c1^2-b1^2)/(2*a1*c1)));
T_Hip = F1*L1;
